simulink model "exp2_bilateral_nodelay_stg1"  (R2025a)
settings: Solver=ode4  StartTime=0.0  StopTime=10.0  FixedStep=1e-4  RelTol=1e-3
undefined symbols (not defined in the file or in its folder): b_eq, Bc, I_eq, k_eq, Kc, r_h, r_m, r_s, vM0, vS0, xM0, xS0
settings Model: Creator=ekaitz  LastModifiedBy=ekaitz

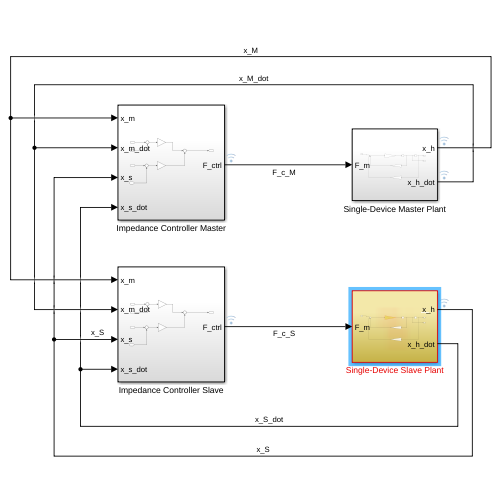
[thumbnail: Simulink's stored preview of the top-level diagram]
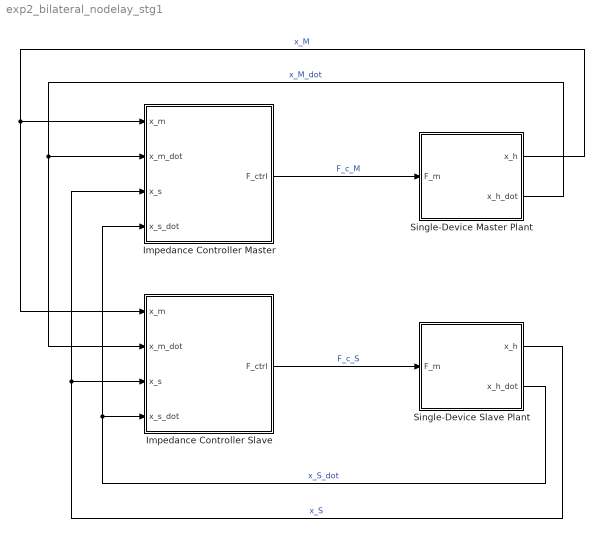
== system exp2_bilateral_nodelay_stg1 ==
  Impedance Controller Master : Subsystem
  Impedance Controller Slave : Subsystem
  Single-Device Master Plant : Subsystem
  Single-Device Slave Plant : Subsystem
  wires:
  Single-Device Slave Plant/2(x_h_dot) -> Impedance Controller Slave/4(x_s_dot), Impedance Controller Master/4(x_s_dot)  "x_S_dot"
  Single-Device Master Plant/2(x_h_dot) -> Impedance Controller Master/2(x_m_dot), Impedance Controller Slave/2(x_m_dot)  "x_M_dot"
  Single-Device Slave Plant/1(x_h) -> Impedance Controller Slave/3(x_s), Impedance Controller Master/3(x_s)  "x_S"
  Impedance Controller Master/1(F_ctrl) -> Single-Device Master Plant/1(F_m)  "F_c_M"
  Single-Device Master Plant/1(x_h) -> Impedance Controller Master/1(x_m), Impedance Controller Slave/1(x_m)  "x_M"
  Impedance Controller Slave/1(F_ctrl) -> Single-Device Slave Plant/1(F_m)  "F_c_S"

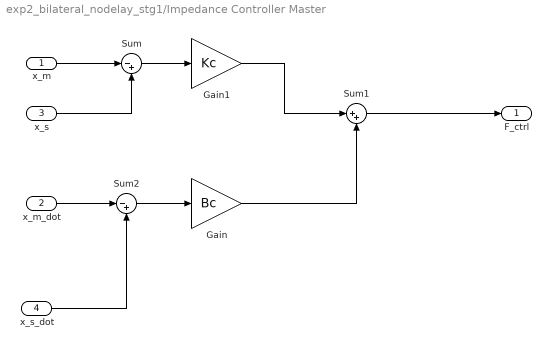
== system exp2_bilateral_nodelay_stg1/Impedance Controller Master ==
  x_m : Inport
  x_m_dot : Inport  Port=2
  x_s : Inport  Port=3
  x_s_dot : Inport  Port=4
  Gain : Gain  Gain=Bc
  Gain1 : Gain  Gain=Kc
  Sum : Sum  Inputs=|-+
  Sum1 : Sum  Inputs=|++
  Sum2 : Sum  Inputs=|-+
  F_ctrl : Outport
  wires:
  x_m/1 -> Sum/1
  Sum/1 -> Gain1/1
  Gain1/1 -> Sum1/1
  Gain/1 -> Sum1/2
  x_s/1 -> Sum/2
  x_m_dot/1 -> Sum2/1
  x_s_dot/1 -> Sum2/2
  Sum2/1 -> Gain/1
  Sum1/1 -> F_ctrl/1

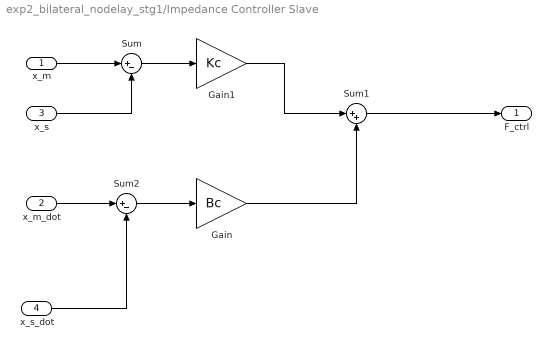
== system exp2_bilateral_nodelay_stg1/Impedance Controller Slave ==
  x_m : Inport
  x_m_dot : Inport  Port=2
  x_s : Inport  Port=3
  x_s_dot : Inport  Port=4
  Gain : Gain  Gain=Bc
  Gain1 : Gain  Gain=Kc
  Sum : Sum  Inputs=|+-
  Sum1 : Sum  Inputs=|++
  Sum2 : Sum  Inputs=|+-
  F_ctrl : Outport
  wires:
  x_m/1 -> Sum/1
  Sum/1 -> Gain1/1
  Gain1/1 -> Sum1/1
  Gain/1 -> Sum1/2
  x_s/1 -> Sum/2
  x_m_dot/1 -> Sum2/1
  x_s_dot/1 -> Sum2/2
  Sum2/1 -> Gain/1
  Sum1/1 -> F_ctrl/1

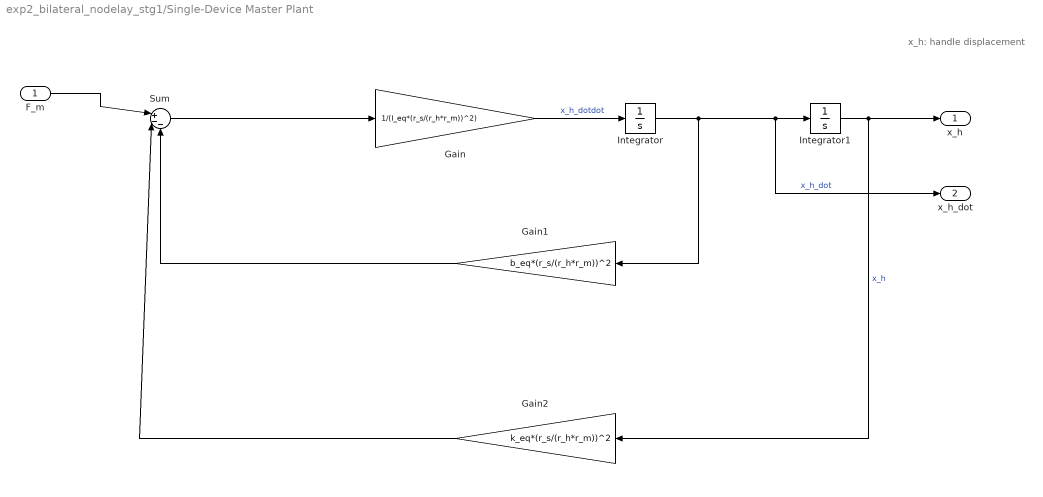
== system exp2_bilateral_nodelay_stg1/Single-Device Master Plant ==
  note: x_h: handle displacement
  F_m : Inport
  Gain : Gain  Gain=1/(I_eq*(r_s/(r_h*r_m))^2)
  Gain1 : Gain  Gain=b_eq*(r_s/(r_h*r_m))^2
  Gain2 : Gain  Gain=k_eq*(r_s/(r_h*r_m))^2
  Integrator : Integrator  InitialCondition=vM0
  Integrator1 : Integrator  InitialCondition=xM0
  Sum : Sum  Inputs=|+--
  x_h : Outport
  x_h_dot : Outport  Port=2
  wires:
  Gain2/1 -> Sum/2
  Gain/1 -> Integrator/1  "x_h_dotdot"
  F_m/1 -> Sum/1
  Integrator1/1 -> x_h/1, Gain2/1  "x_h"
  Gain1/1 -> Sum/3
  Sum/1 -> Gain/1
  Integrator/1 -> Gain1/1, x_h_dot/1, Integrator1/1  "x_h_dot"

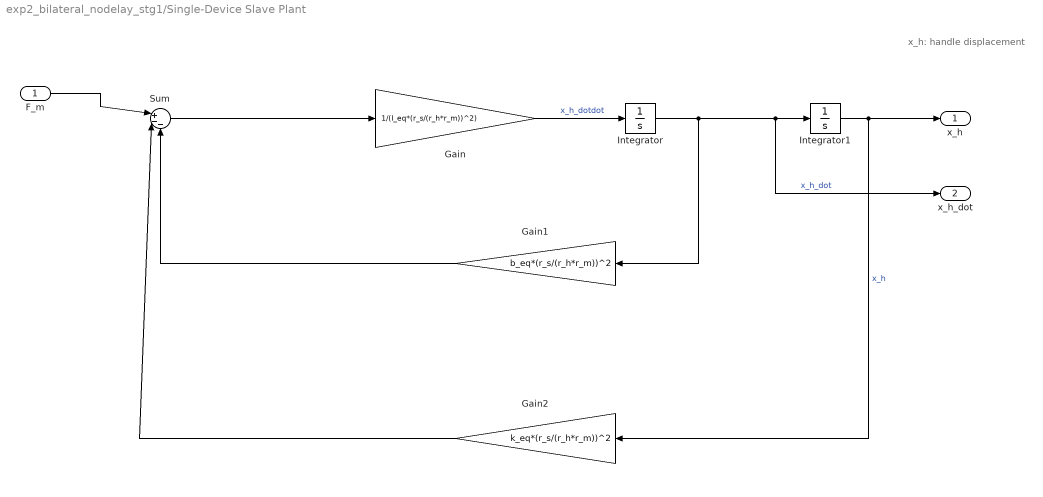
== system exp2_bilateral_nodelay_stg1/Single-Device Slave Plant ==
  note: x_h: handle displacement
  F_m : Inport
  Gain : Gain  Gain=1/(I_eq*(r_s/(r_h*r_m))^2)
  Gain1 : Gain  Gain=b_eq*(r_s/(r_h*r_m))^2
  Gain2 : Gain  Gain=k_eq*(r_s/(r_h*r_m))^2
  Integrator : Integrator  InitialCondition=vS0
  Integrator1 : Integrator  InitialCondition=xS0
  Sum : Sum  Inputs=|+--
  x_h : Outport
  x_h_dot : Outport  Port=2
  wires:
  Gain2/1 -> Sum/2
  Gain/1 -> Integrator/1  "x_h_dotdot"
  F_m/1 -> Sum/1
  Integrator1/1 -> x_h/1, Gain2/1  "x_h"
  Gain1/1 -> Sum/3
  Sum/1 -> Gain/1
  Integrator/1 -> Gain1/1, x_h_dot/1, Integrator1/1  "x_h_dot"
